simulink model "SensAdapt"  (R2013a)
settings: Solver=FixedStepDiscrete  SolverMode=SingleTasking  StartTime=0.0  StopTime=inf  FixedStep=0.01  RelTol=1e-3
libraries: simulink x1
settings Model: Creator=Beny  LastModifiedBy=User
settings DataIOCC: SaveOutput=off  SignalLogging=off  DSMLogging=off  SaveTime=off
settings OptimizationCC: ConditionallyExecuteInputs=off  InlineParams=on  InlineInvariantSignals=on  EnhancedBackFolding=on  BooleansAsBitfields=on  RollThreshold=3  StateBitsets=on  DataBitsets=on  InitFltsAndDblsToZero=on  OptimizeModelRefInitCode=on  LifeSpan=Inf
settings DebuggingCC: SignalInfNanChecking=error  SignalRangeChecking=error  ReadBeforeWriteMsg=EnableAllAsError  WriteAfterWriteMsg=EnableAllAsError  WriteAfterReadMsg=EnableAllAsError  SaveWithParameterizedLinksMsg=error  UnderspecifiedInitializationDetection=Simplified  DiscreteInheritContinuousMsg=error  MultiTaskDSMMsg=warning  SingleTaskRateTransMsg=warning  TasksWithSamePriorityMsg=none  SigSpecEnsureSampleTimeMsg=error  CheckMatrixSingularityMsg=error  IntegerOverflowMsg=error  ParameterUnderflowMsg=error  ParameterPrecisionLossMsg=error  ParameterTunabilityLossMsg=error  FixptConstOverflowMsg=warning  UnderSpecifiedDataTypeMsg=error  UnnecessaryDatatypeConvMsg=warning  VectorMatrixConversionMsg=error  FcnCallInpInsideContextMsg=EnableAllAsWarning  UnconnectedInputMsg=error  UnconnectedOutputMsg=error  UnconnectedLineMsg=error  UniqueDataStoreMsg=error  BusObjectLabelMismatch=error  RootOutportRequireBusObject=error  ModelReferenceIOMsg=error  ModelReferenceIOMismatchMessage=error  ModelReferenceCSMismatchMessage=warning  ModelReferenceDataLoggingMessage=error  StrictBusMsg=ErrorOnBusTreatedAsVector  SFUnexpectedBacktrackingDiag=error  SFInvalidInputDataAccessInChartInitDiag=error  SFNoUnconditionalDefaultTransitionDiag=error  SFTransitionOutsideNaturalParentDiag=error
settings HardwareCC: ProdLargestAtomicInteger=Long  ProdLargestAtomicFloat=Double  ProdEndianess=LittleEndian  ProdHWDeviceType=ARM Compatible->ARM Cortex
settings ModelReferenceCC: ModelReferenceNumInstancesAllowed=Single  ModelReferencePassRootInputsByReference=off
settings RTWCC: SystemTargetFile=ert.tlc  GenCodeOnly=on  TemplateMakefile=ert_default_tmf  Description=Embedded Coder  GenerateReport=on  TLCAssert=on  ProcessScript=ert_make_rtw_hook  IncludeHyperlinkInReport=on  LaunchReport=on  GenerateTraceInfo=on  GenerateTraceReport=on  GenerateTraceReportSl=on  GenerateTraceReportSf=on  GenerateTraceReportEml=on
settings CodeAppCC: ForceParamTrailComments=on  IgnoreCustomStorageClasses=off  IgnoreTestpoints=on  MaxIdLength=64  SimulinkDataObjDesc=on  SFDataObjDesc=on  MangleLength=4  CustomSymbolStrType=$N$R$M  CustomSymbolStrFcnArg=rtu_$I$N$M  DefineNamingRule=UpperCase  InsertBlockDesc=on  MATLABSourceComments=on  InternalIdentifier=Classic  ReqsInCode=on
settings ERTTargetCC: CodeReplacementLibrary=C89/C90 (ANSI)  IncludeMdlTerminateFcn=off  SuppressErrorStatus=on  ParenthesesLevel=Maximum  ERTCustomFileTemplate=example_file_process.tlc  PreserveExpressionOrder=on  PreserveIfCondition=on  ConvertIfToSwitch=on

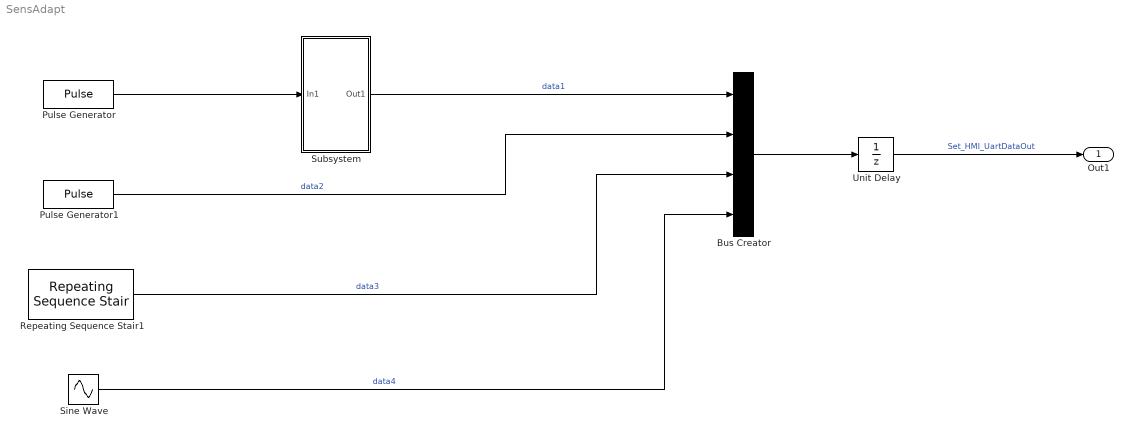
== system SensAdapt ==
  Bus Creator : BusCreator  OutDataTypeStr=Bus: UART_tstDataDisplayed  NonVirtualBus=on
  Pulse Generator : DiscretePulseGenerator  Period=1300  PulseWidth=650  SampleTime=0.01
  Pulse Generator1 : DiscretePulseGenerator  Period=1300  PulseWidth=650  SampleTime=0.01
  Repeating Sequence Stair1 : simulink/Sources/Repeating Sequence Stair  OutValues=[0.123 -0.321 1.45 -2.21 24.456 -54.987 -2134.876 0 4567.987].'  tsamp=-1  OutMin=[]  OutMax=[]  OutDataTypeStr=double  OutputDataTypeScalingMode=double  OutDataType=fixdt(0,8)  ConRadixGroup=Best Precision: Vector-wise  OutScaling=2^-12
  Sine Wave : Sin  SineType=Sample based  Amplitude=2  Samples=100  SampleTime=0.01
  Subsystem : Subsystem
  Unit Delay : UnitDelay  SampleTime=-1
  Out1 : Outport  OutDataTypeStr=Bus: UART_tstDataDisplayed  PortDimensions=1  BusOutputAsStruct=on
  wires:
  Subsystem/1(Out1) -> Bus Creator/1  "data1"
  Bus Creator/1 -> Unit Delay/1
  Pulse Generator1/1 -> Bus Creator/2  "data2"
  Pulse Generator/1 -> Subsystem/1(In1)
  Repeating Sequence Stair1/1 -> Bus Creator/3  "data3"
  Sine Wave/1 -> Bus Creator/4  "data4"
  Unit Delay/1 -> Out1/1  "Set_HMI_UartDataOut"

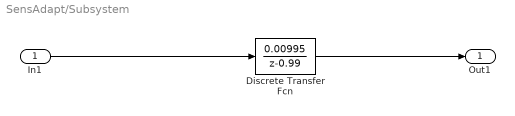
== system SensAdapt/Subsystem ==
  In1 : Inport
  Discrete Transfer Fcn : DiscreteTransferFcn  Numerator=[0.00995]  Denominator=[1 -0.99]
  Out1 : Outport  OutDataTypeStr=double
  wires:
  In1/1 -> Discrete Transfer Fcn/1
  Discrete Transfer Fcn/1 -> Out1/1
